simulink subsystem "code_converter"  (R2020a)
settings: Solver=VariableStepAuto  StartTime=0.0  StopTime=10.0  RelTol=1e-3
settings Model: Creator=upattacini  LastModifiedBy=upattacini

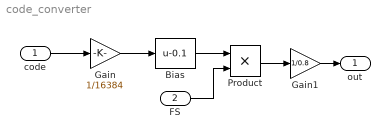
== system code_converter ==
  code : Inport
  FS : Inport  Port=2
  Bias : Bias  Bias=-0.1
  Gain : Gain  Gain=1/16384
  Gain1 : Gain  Gain=1/0.8
  Product : Product
  out : Outport
  wires:
  FS/1 -> Product/2
  Product/1 -> Gain1/1
  Bias/1 -> Product/1
  Gain1/1 -> out/1
  code/1 -> Gain/1
  Gain/1 -> Bias/1
